simulink model "Exercise1"  (R2020a)
settings: Solver=VariableStepAuto  StartTime=0.0  StopTime=inf  RelTol=1e-3
libraries: library_plc2simulink x13
settings Model: EnablePacing=on  Creator=Moritz  LastModifiedBy=Moritz

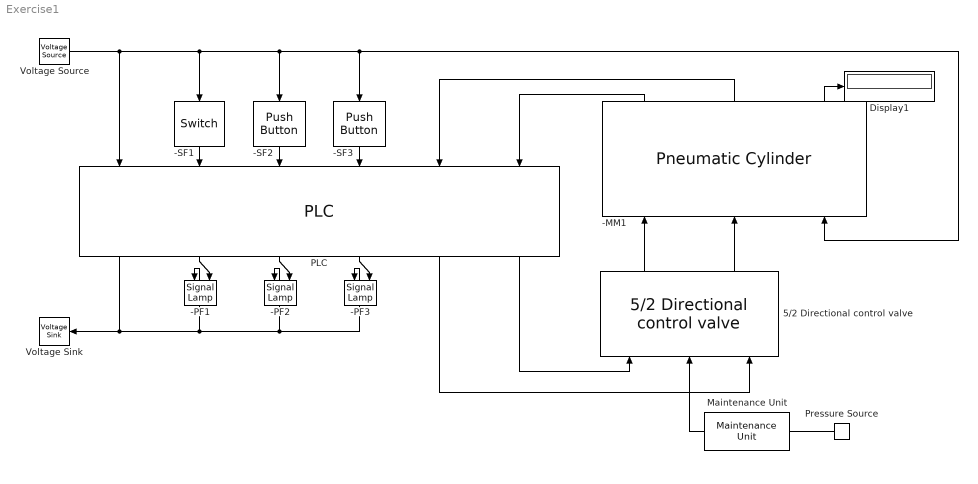
== system Exercise1 ==
  -MM1 : library_plc2simulink/Pneumatic Cylinder  minPos=0  maxPos=100  pistonSpeed=50  currentPos=7.5  updateIcon=0.1
  -PF1 : library_plc2simulink/Signal Lamp  Value=on  updateTime=0.1  colorOn=[0.2,1,0.2]  colorOff=[1,1,1]
  -PF2 : library_plc2simulink/Signal Lamp  Value=off  updateTime=0.1  colorOn=[0.2,1,0.2]  colorOff=[1,1,1]
  -PF3 : library_plc2simulink/Signal Lamp  Value=on  updateTime=0.1  colorOn=[0.2,1,0.2]  colorOff=[1,1,1]
  -SF1 : library_plc2simulink/Switch  Gain=0  Multiplication=Element-wise(K.*u)  ParamMin=[]  ParamMax=[]  OutMin=[]  OutMax=[]  SampleTime=-1
  -SF2 : library_plc2simulink/Push Button  deactTime=0.3  StateOn=0
  -SF3 : library_plc2simulink/Push Button  deactTime=0.3  StateOn=0
  5/2 Directional control valve : library_plc2simulink/5//2 Directional control valve  updateIcon=0.1  state=1
  Display1 : Display
  Maintenance Unit : library_plc2simulink/Maintenance Unit  pressure=1
  PLC : library_plc2simulink/PLC  instanceName=SPS1  numInputs=5  numOutputs=5  timeStep=0.05  externalSupplyVoltage=on
  Pressure Source : library_plc2simulink/Pressure Source  pressure=5
  Voltage Sink : library_plc2simulink/Voltage Sink
  Voltage Source : library_plc2simulink/Voltage Source  voltage=24
  wires:
  -MM1/3 -> Display1/1
  Pressure Source/1 -> Maintenance Unit/1
  Maintenance Unit/1 -> 5/2 Directional control valve/2
  5/2 Directional control valve/1 -> -MM1/1
  5/2 Directional control valve/2 -> -MM1/2
  -SF3/1 -> PLC/4
  Voltage Source/1 -> -MM1/3, -SF3/1, -SF2/1, -SF1/1, PLC/1
  PLC/3 -> -PF2/1
  -SF1/1 -> PLC/2
  -SF2/1 -> PLC/3
  -MM1/1 -> PLC/6
  -MM1/2 -> PLC/5
  PLC/1 -> -PF3/2, -PF2/2, -PF1/2, Voltage Sink/1
  PLC/2 -> -PF1/1
  PLC/6 -> 5/2 Directional control valve/1
  PLC/5 -> 5/2 Directional control valve/3
  PLC/4 -> -PF3/1
